simulink library "MOT_lib"  (R2015a)
settings: Solver=ode45  StartTime=0.0  StopTime=10.0  RelTol=1e-3
undefined symbols (not defined in the file or in its folder): MOT, motor_data
libraries: simulink x1
settings Model: Creator=Andrew  LastModifiedBy=Andrew

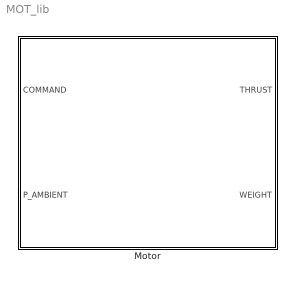
== system MOT_lib ==
  Motor : Subsystem

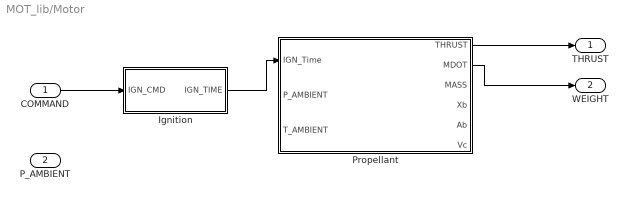
== system MOT_lib/Motor ==
  COMMAND : Inport
  P_AMBIENT : Inport  Port=2
  Ignition : Subsystem
  Propellant : Subsystem
  THRUST : Outport
  WEIGHT : Outport  Port=2
  wires:
  COMMAND/1 -> Ignition/1(IGN_CMD)
  Ignition/1(IGN_TIME) -> Propellant/1(IGN_Time)
  Propellant/1(THRUST) -> THRUST/1
  Propellant/2(MDOT) -> WEIGHT/1

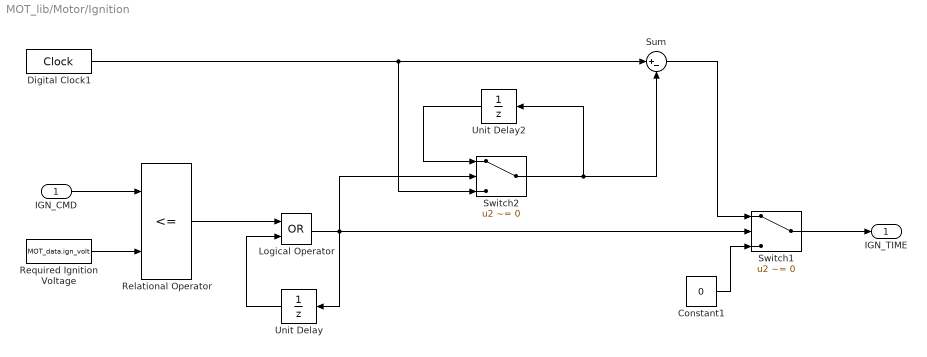
== system MOT_lib/Motor/Ignition ==
  IGN_CMD : Inport
  Constant1 : Constant  Value=0
  Digital Clock1 : DigitalClock  SampleTime=0.0025
  Logical Operator : Logic  Operator=OR  AllPortsSameDT=off  OutDataTypeStr=boolean
  Relational Operator : RelationalOperator  Operator=<=  OutDataTypeStr=boolean
  Required Ignition Voltage : FromWorkspace  VariableName=MOT_data.ign_volt  SampleTime=0
  Sum : Sum  Inputs=|+-
  Switch1 : Switch  Criteria=u2 ~= 0
  Switch2 : Switch  Criteria=u2 ~= 0
  Unit Delay : UnitDelay  SampleTime=-1
  Unit Delay2 : UnitDelay  SampleTime=-1
  IGN_TIME : Outport
  wires:
  IGN_CMD/1 -> Relational Operator/1
  Required Ignition Voltage/1 -> Relational Operator/2
  Relational Operator/1 -> Logical Operator/1
  Unit Delay/1 -> Logical Operator/2
  Constant1/1 -> Switch1/3
  Logical Operator/1 -> Switch1/2, Unit Delay/1, Switch2/2
  Digital Clock1/1 -> Switch2/3, Sum/1
  Sum/1 -> Switch1/1
  Switch1/1 -> IGN_TIME/1
  Switch2/1 -> Unit Delay2/1, Sum/2
  Unit Delay2/1 -> Switch2/1

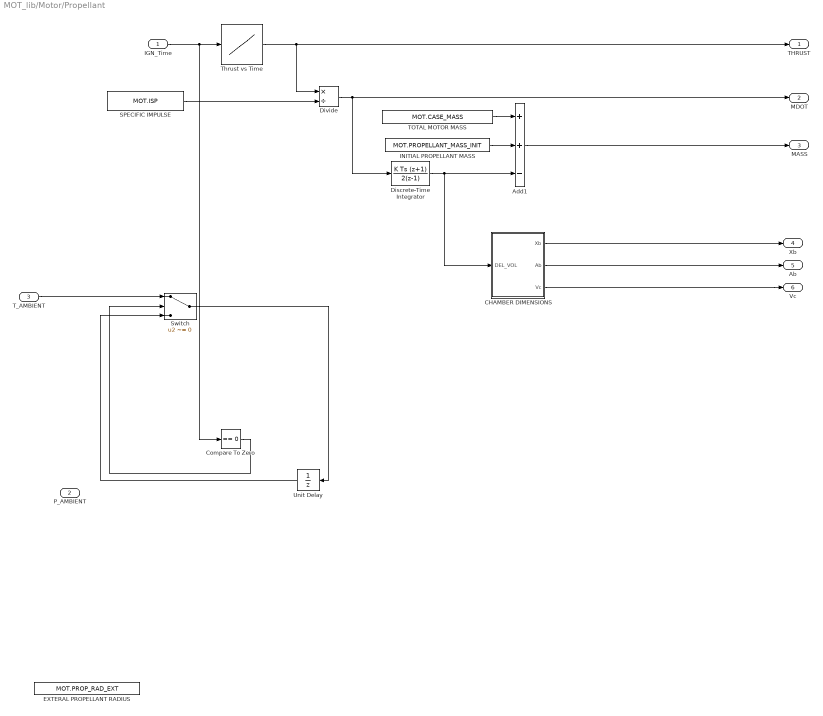
== system MOT_lib/Motor/Propellant ==
  IGN_Time : Inport
  P_AMBIENT : Inport  Port=2
  T_AMBIENT : Inport  Port=3
  Add1 : Sum  Inputs=++-
  CHAMBER DIMENSIONS : Subsystem
  Compare To Zero : simulink/Logic and Bit Operations/Compare To Zero  relop===  OutDataTypeStr=boolean
  Discrete-Time Integrator : DiscreteIntegrator  IntegratorMethod=Integration: Trapezoidal  InitialConditionSetting=State (most efficient)  SampleTime=-1
  Divide : Product  Inputs=*/
  EXTERAL PROPELLANT RADIUS : Constant  Value=MOT.PROP_RAD_EXT
  INITIAL PROPELLANT MASS : Constant  Value=MOT.PROPELLANT_MASS_INIT
  SPECIFIC IMPULSE : Constant  Value=MOT.ISP
  Switch : Switch  Criteria=u2 ~= 0
  TOTAL MOTOR MASS : Constant  Value=MOT.CASE_MASS
  Thrust vs Time : Lookup_n-D  NumberOfTableDimensions=1  BreakpointsForDimension1=motor_data.time  Table=motor_data.thrust  InternalRulePriority=Speed  RndMeth=Simplest  InputSameDT=on
  Unit Delay : UnitDelay  SampleTime=-1
  THRUST : Outport
  MDOT : Outport  Port=2
  MASS : Outport  Port=3
  Xb : Outport  Port=4
  Ab : Outport  Port=5
  Vc : Outport  Port=6
  wires:
  IGN_Time/1 -> Compare To Zero/1, Thrust vs Time/1
  Thrust vs Time/1 -> Divide/1, THRUST/1
  T_AMBIENT/1 -> Switch/1
  Compare To Zero/1 -> Switch/2
  Switch/1 -> Unit Delay/1
  Unit Delay/1 -> Switch/3
  SPECIFIC IMPULSE/1 -> Divide/2
  Divide/1 -> MDOT/1, Discrete-Time Integrator/1
  INITIAL PROPELLANT MASS/1 -> Add1/2
  Discrete-Time Integrator/1 -> CHAMBER DIMENSIONS/1(DEL_VOL), Add1/3
  TOTAL MOTOR MASS/1 -> Add1/1
  Add1/1 -> MASS/1
  CHAMBER DIMENSIONS/1(Xb) -> Xb/1
  CHAMBER DIMENSIONS/2(Ab) -> Ab/1
  CHAMBER DIMENSIONS/3(Vc) -> Vc/1

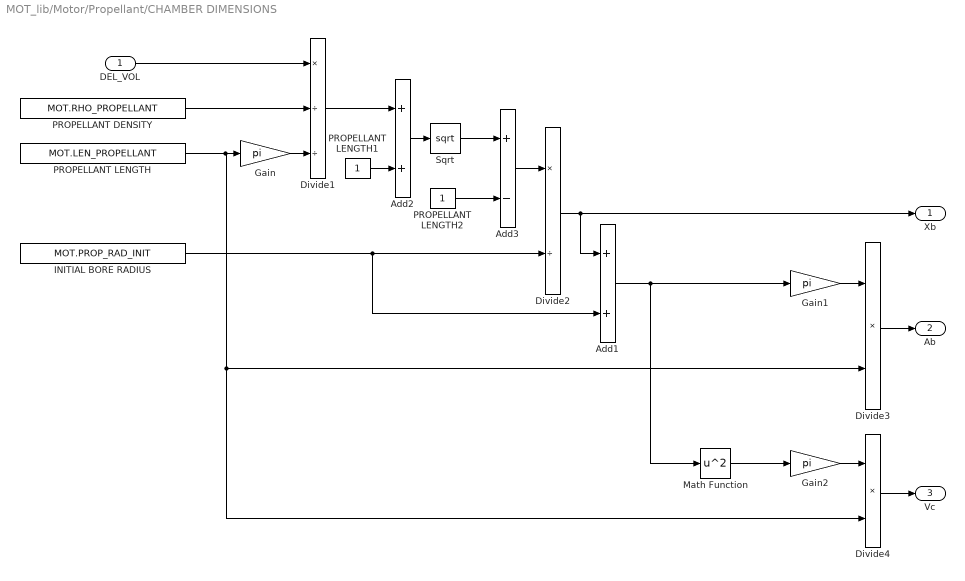
== system MOT_lib/Motor/Propellant/CHAMBER DIMENSIONS ==
  DEL_VOL : Inport
  Add1 : Sum
  Add2 : Sum
  Add3 : Sum  Inputs=+-
  Divide1 : Product  Inputs=*//
  Divide2 : Product  Inputs=*/
  Divide3 : Product  Inputs=**
  Divide4 : Product  Inputs=**
  Gain : Gain  Gain=pi
  Gain1 : Gain  Gain=pi
  Gain2 : Gain  Gain=pi
  INITIAL BORE RADIUS : Constant  Value=MOT.PROP_RAD_INIT
  Math Function : Math  Operator=square  SaturateOnIntegerOverflow=on
  PROPELLANT DENSITY : Constant  Value=MOT.RHO_PROPELLANT
  PROPELLANT LENGTH : Constant  Value=MOT.LEN_PROPELLANT
  PROPELLANT LENGTH1 : Constant
  PROPELLANT LENGTH2 : Constant
  Sqrt : Sqrt  SaturateOnIntegerOverflow=on
  Xb : Outport
  Ab : Outport  Port=2
  Vc : Outport  Port=3
  wires:
  PROPELLANT DENSITY/1 -> Divide1/2
  Gain/1 -> Divide1/3
  Divide1/1 -> Add2/1
  Add2/1 -> Sqrt/1
  Sqrt/1 -> Add3/1
  PROPELLANT LENGTH2/1 -> Add3/2
  PROPELLANT LENGTH1/1 -> Add2/2
  PROPELLANT LENGTH/1 -> Divide3/2, Divide4/2, Gain/1
  DEL_VOL/1 -> Divide1/1
  Add3/1 -> Divide2/1
  Divide2/1 -> Xb/1, Add1/1
  INITIAL BORE RADIUS/1 -> Add1/2, Divide2/2
  Add1/1 -> Gain1/1, Math Function/1
  Gain1/1 -> Divide3/1
  Divide3/1 -> Ab/1
  Divide4/1 -> Vc/1
  Gain2/1 -> Divide4/1
  Math Function/1 -> Gain2/1
